simulink model "newSensorFinal"  (R2021a)
settings: Solver=FixedStepAuto  StartTime=0.0  StopTime=20.0  RelTol=1e-3  EnableMultiTasking=on
libraries: raspberrypiCommlib x6, raspberrypiBasiclib x4
settings Model: Creator=Administrator  LastModifiedBy=pouria
settings SolverCC: PositivePriorityOrder=on  AutoInsertRateTranBlk=on
settings OptimizationCC: EnhancedBackFolding=on  PassReuseOutputArgsAs=Individual arguments  ZeroExternalMemoryAtStartup=off  ZeroInternalMemoryAtStartup=off  MaxStackSize=64  OptimizeBlockOrder=speed  DifferentSizesBufferReuse=on  OptimizationCustomize=off  EfficientTunableParamExpr=on
settings DebuggingCC: ParameterTunabilityLossMsg=error
settings HardwareCC: ProdBitPerPointer=32  ProdBitPerSizeT=32  ProdBitPerPtrDiffT=32  ProdLargestAtomicInteger=Long  ProdLargestAtomicFloat=Double  ProdWordSize=32  ProdLongLongMode=on  ProdHWDeviceType=ARM Compatible->ARM Cortex
settings RTWCC: SystemTargetFile=ert.tlc  HardwareBoard=Raspberry Pi  TLCOptions="-aInlineSetEventsForThisBaseRateFcn=TLC_FALSE -aSuppressMultiTaskScheduler=TLC_FALSE  -aRateBasedStepFcn=0"  TemplateMakefile=ert_default_tmf  Toolchain=GNU GCC Embedded Linux  BuildConfiguration=Faster Runs
settings CodeAppCC: ForceParamTrailComments=on  IgnoreCustomStorageClasses=off  OperatorAnnotations=on  SimulinkDataObjDesc=on  SFDataObjDesc=on  InsertBlockDesc=on
settings ERTTargetCC: SupportContinuousTime=on  SupportVariableSizeSignals=on  ExtModeTransport=2  ExtModeStaticAlloc=on  ExtModeMexFile=ext_xcp  ExtModeIntrfLevel=Level2 - Open

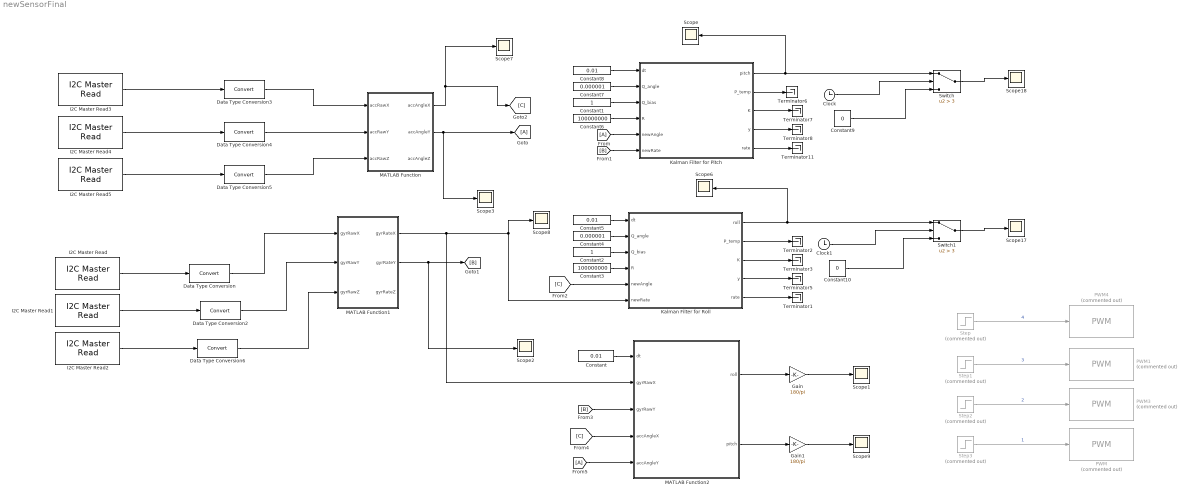
== system newSensorFinal ==
  Clock : Clock
  Clock1 : Clock
  Constant : Constant  Value=0.01
  Constant1 : Constant  SampleTime=0.01
  Constant10 : Constant  Value=0
  Constant2 : Constant  SampleTime=0.01
  Constant3 : Constant  Value=100000000  SampleTime=0.01
  Constant4 : Constant  Value=0.000001  SampleTime=0.01
  Constant5 : Constant  Value=0.01  SampleTime=0.01
  Constant6 : Constant  Value=100000000  SampleTime=0.01
  Constant7 : Constant  Value=0.000001  SampleTime=0.01
  Constant8 : Constant  Value=0.01  SampleTime=0.01
  Constant9 : Constant  Value=0
  Data Type Conversion{,2..6} (6 alike) : DataTypeConversion
  Gain : Gain  Gain=180/pi
  Gain1 : Gain  Gain=180/pi
  I2C Master Read : raspberrypiCommlib/I2C Master Read  BoardProperty=Pi 3 Model B+  Mode=Master  SlaveAddress="hex2dec(\"0x68\")"  SlaveByteOrder=BigEndian  Direction=Receiver  RegisterAddressMode=on  RegisterAddress=67  SlaveDataType=int16  DataLength=1  NoAck=off  RepeatedStart=off  OutputStatus=off  SampleTime=0.01
      settings: SourceProductBaseCode=RASPPI
  I2C Master Read1 : raspberrypiCommlib/I2C Master Read  BoardProperty=Pi 3 Model B+  Mode=Master  SlaveAddress="hex2dec(\"0x68\")"  SlaveByteOrder=BigEndian  Direction=Receiver  RegisterAddressMode=on  RegisterAddress=69  SlaveDataType=int16  DataLength=1  NoAck=off  RepeatedStart=off  OutputStatus=off  SampleTime=0.01
      settings: SourceProductBaseCode=RASPPI
  I2C Master Read2 : raspberrypiCommlib/I2C Master Read  BoardProperty=Pi 3 Model B+  Mode=Master  SlaveAddress="hex2dec(\"0x68\")"  SlaveByteOrder=BigEndian  Direction=Receiver  RegisterAddressMode=on  RegisterAddress=71  SlaveDataType=int16  DataLength=1  NoAck=off  RepeatedStart=off  OutputStatus=off  SampleTime=0.01
      settings: SourceProductBaseCode=RASPPI
  I2C Master Read3 : raspberrypiCommlib/I2C Master Read  BoardProperty=Pi 3 Model B+  Mode=Master  SlaveAddress="hex2dec(\"0x68\")"  SlaveByteOrder=BigEndian  Direction=Receiver  RegisterAddressMode=on  RegisterAddress=59  SlaveDataType=int16  DataLength=1  NoAck=off  RepeatedStart=off  OutputStatus=off  SampleTime=0.01
      settings: SourceProductBaseCode=RASPPI
  I2C Master Read4 : raspberrypiCommlib/I2C Master Read  BoardProperty=Pi 3 Model B+  Mode=Master  SlaveAddress="hex2dec(\"0x68\")"  SlaveByteOrder=BigEndian  Direction=Receiver  RegisterAddressMode=on  RegisterAddress=61  SlaveDataType=int16  DataLength=1  NoAck=off  RepeatedStart=off  OutputStatus=off  SampleTime=0.01
      settings: SourceProductBaseCode=RASPPI
  I2C Master Read5 : raspberrypiCommlib/I2C Master Read  BoardProperty=Pi 3 Model B+  Mode=Master  SlaveAddress="hex2dec(\"0x68\")"  SlaveByteOrder=BigEndian  Direction=Receiver  RegisterAddressMode=on  RegisterAddress=63  SlaveDataType=int16  DataLength=1  NoAck=off  RepeatedStart=off  OutputStatus=off  SampleTime=0.01
      settings: SourceProductBaseCode=RASPPI
  Kalman Filter for Pitch : MATLAB Function  TreatAsAtomicUnit=on
  Kalman Filter for Roll : MATLAB Function  TreatAsAtomicUnit=on
  MATLAB Function : MATLAB Function  TreatAsAtomicUnit=on
  MATLAB Function1 : MATLAB Function  TreatAsAtomicUnit=on
  MATLAB Function2 : MATLAB Function  TreatAsAtomicUnit=on
  PWM : raspberrypiBasiclib/PWM  Commented=on  board=Pi 3 Model B+  Pin_=21  Frequency=400  blockPlatform=Raspberry Pi
      settings: SourceProductBaseCode=RASPPI
  PWM1 : raspberrypiBasiclib/PWM  Commented=on  board=Pi 3 Model B+  Pin_=20  Frequency=400  blockPlatform=Raspberry Pi
      settings: SourceProductBaseCode=RASPPI
  PWM3 : raspberrypiBasiclib/PWM  Commented=on  board=Pi 3 Model B+  Pin_=16  Frequency=400  blockPlatform=Raspberry Pi
      settings: SourceProductBaseCode=RASPPI
  PWM4 : raspberrypiBasiclib/PWM  Commented=on  board=Pi 3 Model B+  Pin_=19  Frequency=400  blockPlatform=Raspberry Pi
      settings: SourceProductBaseCode=RASPPI
  Scope{,1..3,6..9,17..18} (10 alike) : Scope
  Step{,1..3} (4 alike) : Step  Commented=on  Time=5  Before=0.3  After=0.4  SampleTime=0.01
  Switch : Switch  Criteria=u2 > Threshold  Threshold=3
  Switch1 : Switch  Criteria=u2 > Threshold  Threshold=3
  Terminator{1..3,5..8,11} (8 alike) : Terminator
  wires:
  I2C Master Read3/1 -> Data Type Conversion3/1
  I2C Master Read4/1 -> Data Type Conversion4/1
  I2C Master Read5/1 -> Data Type Conversion5/1
  Data Type Conversion3/1 -> MATLAB Function/1(accRawX)
  Data Type Conversion4/1 -> MATLAB Function/2(accRawY)
  Data Type Conversion5/1 -> MATLAB Function/3(accRawZ)
  Data Type Conversion/1 -> MATLAB Function1/1(gyrRawX)
  Data Type Conversion2/1 -> MATLAB Function1/2(gyrRawY)
  Constant5/1 -> Kalman Filter for Roll/1(dt)
  Constant3/1 -> Kalman Filter for Roll/4(R)
  Constant2/1 -> Kalman Filter for Roll/3(Q_bias)
  Constant4/1 -> Kalman Filter for Roll/2(Q_angle)
  Constant1/1 -> Kalman Filter for Pitch/3(Q_bias)
  Constant8/1 -> Kalman Filter for Pitch/1(dt)
  Constant6/1 -> Kalman Filter for Pitch/4(R)
  Constant7/1 -> Kalman Filter for Pitch/2(Q_angle)
  [B] -> Kalman Filter for Pitch/6(newRate)
  [A] -> Kalman Filter for Pitch/5(newAngle)
  [C] -> Kalman Filter for Roll/5(newAngle)
  Kalman Filter for Pitch/2(P_temp) -> Terminator6/1
  Kalman Filter for Pitch/3(K) -> Terminator7/1
  Kalman Filter for Pitch/4(y) -> Terminator8/1
  Kalman Filter for Pitch/5(rate) -> Terminator11/1
  Kalman Filter for Roll/2(P_temp) -> Terminator2/1
  Kalman Filter for Roll/4(y) -> Terminator5/1
  Kalman Filter for Roll/5(rate) -> Terminator1/1
  Kalman Filter for Roll/3(K) -> Terminator3/1
  I2C Master Read2/1 -> Data Type Conversion6/1
  I2C Master Read1/1 -> Data Type Conversion2/1
  I2C Master Read/1 -> Data Type Conversion/1
  Clock/1 -> Switch/2
  Constant9/1 -> Switch/3
  Constant10/1 -> Switch1/3
  Clock1/1 -> Switch1/2
  Kalman Filter for Roll/1(roll) -> Scope6/1, Switch1/1
  Kalman Filter for Pitch/1(pitch) -> Scope/1, Switch/1
  Switch/1 -> Scope18/1
  Switch1/1 -> Scope17/1
  Data Type Conversion6/1 -> MATLAB Function1/3(gyrRawZ)
  MATLAB Function/1(accAngleX) -> [C], Scope7/1
  MATLAB Function/2(accAngleY) -> [A], Scope3/1
  MATLAB Function1/1(gyrRateX) -> MATLAB Function2/2(gyrRawX), Kalman Filter for Roll/6(newRate), Scope8/1
  MATLAB Function1/2(gyrRateY) -> [B], Scope2/1
  Constant/1 -> MATLAB Function2/1(dt)
  [B] -> MATLAB Function2/3(gyrRawY)
  [C] -> MATLAB Function2/4(accAngleX)
  [A] -> MATLAB Function2/5(accAngleY)
  MATLAB Function2/1(roll) -> Gain/1
  MATLAB Function2/2(pitch) -> Gain1/1
  Gain/1 -> Scope1/1
  Gain1/1 -> Scope9/1
  Step/1 -> PWM4/1  "4"
  Step1/1 -> PWM1/1  "3"
  Step2/1 -> PWM3/1  "2"
  Step3/1 -> PWM/1  "1"

== matlab function newSensorFinal/MATLAB Function ==
  data: accRawX input; accAngleX output; accAngleY output; accRawY input; accRawZ input; accAngleZ output
function [accAngleX, accAngleY, accAngleZ] = fcn(accRawX, accRawY, accRawZ)

%Converting the raw accel data from g values to accel about X and Y axis

accAngleX = atan(accRawY/sqrt(power(accRawX,2) + power(accRawZ,2)))*(180/pi);
accAngleY = atan(-1*(accRawX/sqrt(power(accRawY,2) + power(accRawZ,2))))*(180/pi);
accAngleZ = atan(accRawZ/sqrt(power(accRawX,2) + power(accRawZ,2)))*(180/pi);

end

== matlab function newSensorFinal/MATLAB Function1 ==
  data: gyrRawX input; gyrRateX output; gyrRateY output; gyrRawY input; gyrRawZ input; gyrRateZ output
function [gyrRateX, gyrRateY, gyrRateZ] = fcn(gyrRawX, gyrRawY, gyrRawZ)

gyrRateX = gyrRawX/131.0;
gyrRateY = gyrRawY/131.0;
gyrRateZ = gyrRawZ/131.0;

end

== matlab function newSensorFinal/Kalman Filter for Pitch ==
  data: dt input; pitch output; Q_angle input; Q_bias input; R input; newAngle input; newRate input; P_temp output; K output; y output; rate output
function [pitch, P_temp, K, y, rate]  = kalFilterPitch(dt, Q_angle, Q_bias, R, newAngle, newRate)

persistent angle;
persistent P;
persistent bias_p;

%Process Noise Convariance Matrix
Q = [Q_angle 0; 0 Q_bias] * dt;
F = [1  dt; 0 1];
H = [1 0];
% bias = 6.7483;

if isempty(bias_p)
    bias_p = 6.7371;
end

rate = newRate - bias_p;

if isempty(angle); angle = 0;
    
else
    angle = angle + (dt * rate);
end 

pitch = angle;

if isempty(P); P = [0, 0; 0, 0];
else
    P = F*P*F' + Q;
end 
P_temp = P;

S = H*P*H' + R;
K = (P_temp * H')/S;
y = newAngle - pitch; 
pitch = pitch + K(1) * y;
bias_p = bias_p + K(2) * y;
angle = pitch;

I = [1 0; 0 1];
P_temp = (I - K*H)*P_temp;
P = P_temp;

return 


end

== matlab function newSensorFinal/Kalman Filter for Roll ==
  data: dt input; roll output; Q_angle input; Q_bias input; R input; newAngle input; newRate input; P_temp output; K output; y output; rate output
function [roll, P_temp, K, y, rate]  = kalFilterRoll(dt, Q_angle, Q_bias, R, newAngle, newRate)

persistent angle;
persistent P;
persistent bias_r;

%Process Noise Convariance Matrix
Q = [Q_angle 0; 0 Q_bias] * dt;
F = [1  dt; 0 1];
H = [1 0];
% bias = 3.3726;

if isempty(bias_r)
    bias_r = 3.7342;
end

rate = newRate - bias_r;

if isempty(angle); angle = 0;
    
else
    angle = angle + (dt * rate);
end 

roll = angle;

if isempty(P); P = [0, 0; 0, 0];
else
    P = F*P*F' + Q;
end 
P_temp = P;

S = H*P*H' + R;
K = (P_temp * H')/S;
y = newAngle - roll; 
roll = roll + K(1) * y;
bias_r = bias_r + K(2) * y;
angle = roll;

I = [1 0; 0 1];
P_temp = (I - K*H)*P_temp;
P = P_temp;

return 


end

== matlab function newSensorFinal/MATLAB Function2 ==
  data: dt input; roll output; pitch output; gyrRawX input; gyrRawY input; accAngleX input; accAngleY input
function [roll, pitch] = complimentaryF(dt, gyrRawX, gyrRawY, accAngleX, accAngleY)

 gyrAngleX = gyrRawX * dt;
 gyrAngleY = gyrRawY * dt;
 roll = 0.98 * (gyrAngleX) + 0.02 * accAngleX;
 pitch = 0.98 * (gyrAngleY) + 0.02 * accAngleY;
 
end
